simulink model "Main"  (R2020b)
settings: Solver=FixedStepAuto  StartTime=0.0  StopTime=inf  FixedStep=0.010  RelTol=1e-3
libraries: TcSimInterface x1
(part 2 of 2)

== matlab function Main/Split Actor Information ==
  data: plcSignal input; sigCreate output; sigRemove output; acUpOpen output; acUpClose output; acDownOpen output; acDownClose output
function [sigCreate, sigRemove, acUpOpen, acUpClose, acDownOpen, acDownClose] = DeCombineActuators(plcSignal)
    sigCreate = bitget(plcSignal,1);
    sigRemove = bitget(plcSignal,2);
 %   ~ = bitget(plcSignal,3);
%    ~ = bitget(plcSignal,4);

    acDownClose = bitget(plcSignal,5);
    acDownOpen = bitget(plcSignal,6);
    acUpClose = bitget(plcSignal,7);
    acUpOpen = bitget(plcSignal,8);
end

== matlab function Main/Combine Sensor Data ==
  data: sensDown input; combinedSensors output; sensMiddle input; sensUp input
function combinedSensors  = CombineSensors(sensDown, sensMiddle, sensUp)
% 0000_0DMU
sensDown = bitshift(sensDown, 2);
sensMiddle = bitshift(sensMiddle, 1);
sensUp = bitshift(sensUp, 0);



combinedSensors = bitor(sensDown, bitor(sensMiddle,sensUp));
